simulink model "read_scaled_imu"  (R2024a)
settings: Solver=ode4  StartTime=0.0  StopTime=100  FixedStep=sampleTime  RelTol=1e-3
values from neighbouring files (symbols this model uses):
  sampleTime = 1/500    (= 0.002)    [read_imu.m]
undefined symbols (not defined in the file or in its folder): f
libraries: simulink_extras x9, uavmavlinklib x4, instrumentlib x2, aerolibanimutils x1, px4MAVLinkBridgelib x1, mspfiltlib x1, dspstat3 x1
settings Model: Creator=user  LastModifiedBy=user

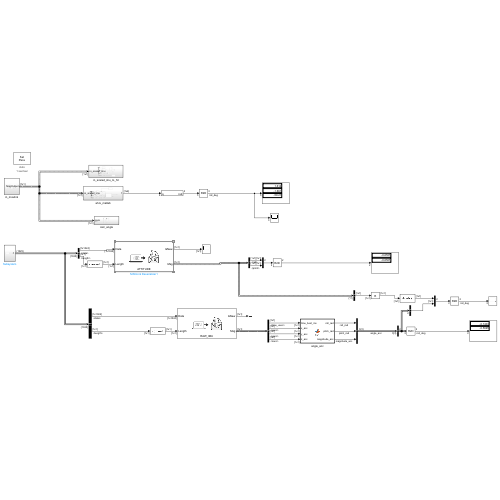
[thumbnail: Simulink's stored preview of the top-level diagram]
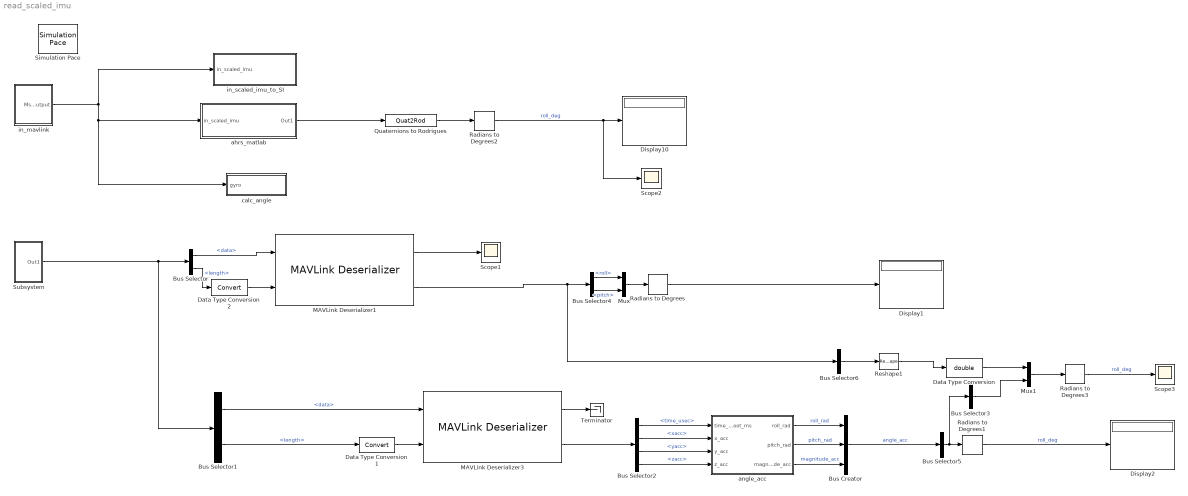
== system read_scaled_imu ==
  Bus Creator : BusCreator  Inputs=3
  Bus Selector : BusSelector  OutputSignals=data,length
  Bus Selector1 : BusSelector  OutputSignals=data,length
  Bus Selector2 : BusSelector  OutputSignals=Payload.time_usec,Payload.xacc,Payload.yacc,Payload.zacc
  Bus Selector3 : BusSelector  OutputSignals=roll_rad  OutputAsBus=on
  Bus Selector4 : BusSelector  OutputSignals=Payload.roll,Payload.pitch
  Bus Selector5 : BusSelector  OutputSignals=roll_rad,pitch_rad  OutputAsBus=on
  Bus Selector6 : BusSelector  OutputSignals=Payload.roll  OutputAsBus=on
  Data Type Conversion : DataTypeConversion  OutDataTypeStr=double  SaturateOnIntegerOverflow=off  RndMeth=Floor
  Data Type Conversion1 : DataTypeConversion  SaturateOnIntegerOverflow=off  RndMeth=Floor
  Data Type Conversion2 : DataTypeConversion  SaturateOnIntegerOverflow=off  RndMeth=Floor
  Display1 : Display
  Display10 : Display
  Display2 : Display
  MAVLink Deserializer1 : uavmavlinklib/MAVLink Deserializer  dialectSource=Select from standard MAVLink dialects  dialect=common.xml  dialectCustom=common.xml  version=2  messageType=ATTITUDE  inputDataLength=on  SystemIDFilter=off  systemID=1  ComponentIDFilter=off  componentID=1  queueMsg=off  queueMsgSize=50  dropNum=off
  MAVLink Deserializer3 : uavmavlinklib/MAVLink Deserializer  dialectSource=Select from standard MAVLink dialects  dialect=common.xml  dialectCustom=common.xml  version=2  messageType=RAW_IMU  inputDataLength=on  SystemIDFilter=off  systemID=1  ComponentIDFilter=off  componentID=1  queueMsg=off  queueMsgSize=50  dropNum=off
  Mux : Mux  Inputs=2
  Mux1 : Mux  Inputs=2
  Quaternions to Rodrigues : Quat2Rod
  Radians to Degrees{,1..3} (4 alike) : simulink_extras/Transformations/Radians to Degrees
  Reshape1 : Reshape  OutputDimensionality=Customize
  Scope1 : Scope
  Scope2 : Scope
  Scope3 : Scope
  Simulation Pace : aerolibanimutils/Simulation Pace  SimulationPace=1  SleepMode=Auto  OutputPaceError=off  SampleTime=sampleTime
  Subsystem : Subsystem
  Terminator : Terminator
  ahrs_matlab : Subsystem
  angle_acc : MATLAB Function  TreatAsAtomicUnit=on
  calc_angle : Subsystem
  in_mavlink : Subsystem
  in_scaled_imu_to_SI : Subsystem
  wires:
  Quaternions to Rodrigues/1 -> Radians to Degrees2/1
  Radians to Degrees2/1 -> Scope2/1, Display10/1  "roll_deg"
  ahrs_matlab/1(Out1) -> Quaternions to Rodrigues/1
  in_mavlink/1(MsgOutput) -> calc_angle/1(gyro), ahrs_matlab/1(in_scaled_imu), in_scaled_imu_to_SI/1(in_scaled_imu)
  Bus Selector4/1 -> Mux/1  "<roll>"
  MAVLink Deserializer1/2 -> Bus Selector6/1, Bus Selector4/1
  Data Type Conversion2/1 -> MAVLink Deserializer1/2
  MAVLink Deserializer1/1 -> Scope1/1
  Bus Selector4/2 -> Mux/2  "<pitch>"
  Mux/1 -> Radians to Degrees/1
  Radians to Degrees/1 -> Display1/1
  Bus Selector/1 -> MAVLink Deserializer1/1  "<data>"
  Bus Selector/2 -> Data Type Conversion2/1  "<length>"
  Data Type Conversion1/1 -> MAVLink Deserializer3/2
  Bus Selector1/2 -> Data Type Conversion1/1  "<length>"
  Bus Selector1/1 -> MAVLink Deserializer3/1  "<data>"
  Subsystem/1(Out1) -> Bus Selector1/1, Bus Selector/1
  angle_acc/3(magnitude_acc) -> Bus Creator/3  "magnitude_acc"
  Radians to Degrees1/1 -> Display2/1  "roll_deg"
  angle_acc/1(roll_rad) -> Bus Creator/1  "roll_rad"
  angle_acc/2(pitch_rad) -> Bus Creator/2  "pitch_rad"
  Bus Creator/1 -> Bus Selector5/1  "angle_acc"
  MAVLink Deserializer3/2 -> Bus Selector2/1
  Bus Selector2/3 -> angle_acc/3(y_acc)  "<yacc>"
  Bus Selector2/2 -> angle_acc/2(x_acc)  "<xacc>"
  Bus Selector5/1 -> Bus Selector3/1, Radians to Degrees1/1
  Bus Selector2/4 -> angle_acc/4(z_acc)  "<zacc>"
  Bus Selector2/1 -> angle_acc/1(time_boot_ms)  "<time_usec>"
  Bus Selector6/1 -> Reshape1/1
  Bus Selector3/1 -> Mux1/2
  Mux1/1 -> Radians to Degrees3/1
  Radians to Degrees3/1 -> Scope3/1  "roll_deg"
  Reshape1/1 -> Data Type Conversion/1
  Data Type Conversion/1 -> Mux1/1
  MAVLink Deserializer3/1 -> Terminator/1

== system read_scaled_imu/Subsystem ==
  Bus Creator : BusCreator  Inputs=2
  MAVLink Bridge Source : px4MAVLinkBridgelib/MAVLink Bridge Source  PixhawkSerialPorttemp=COM7  PixhawkSerialPortManually=COM4  dataLength=1024  FieldTable={ 'UDP', '127.0.0.1', '14550' }  SampleTime=1/50
  Out1 : Outport
  wires:
  MAVLink Bridge Source/2 -> Bus Creator/2  "length"
  MAVLink Bridge Source/1 -> Bus Creator/1  "data"
  Bus Creator/1 -> Out1/1

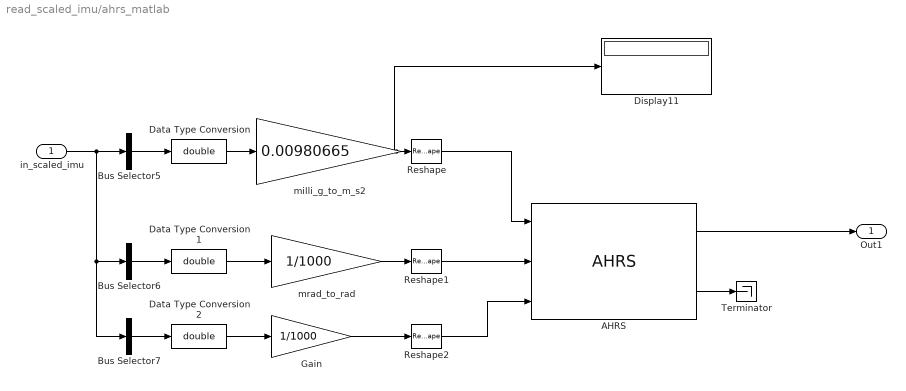
== system read_scaled_imu/ahrs_matlab ==
  in_scaled_imu : Inport
  AHRS : mspfiltlib/AHRS  DispRefFrame=ENU  DecimationFactor=1  InitialProcessNoise=ahrsfilter.defaultProcessNoise  OrientationFormat=quaternion  SimulateUsing=Code generation  AccelerometerNoise=0.0001924722*0+5.11e-6  GyroscopeNoise=9.1385e-5*0+6.86e-8  MagnetometerNoise=0.1e-5  GyroscopeDriftNoise=3.0462e-13*0+1e-8  LinearAccelerationNoise=0.0096236100000000012  MagneticDisturbanceNoise=0.5  LinearAccelerationDecayFactor=0.5*0  MagneticDisturbanceDecayFactor=0.5  ExpectedMagneticFieldStrength=50
  Bus Selector5 : BusSelector  OutputSignals=Payload.xacc,Payload.yacc,Payload.zacc  OutputAsBus=on
  Bus Selector6 : BusSelector  OutputSignals=Payload.xgyro,Payload.ygyro,Payload.zgyro  OutputAsBus=on
  Bus Selector7 : BusSelector  OutputSignals=Payload.xmag,Payload.ymag,Payload.zmag  OutputAsBus=on
  Data Type Conversion : DataTypeConversion  OutDataTypeStr=double  SaturateOnIntegerOverflow=off  RndMeth=Floor
  Data Type Conversion1 : DataTypeConversion  OutDataTypeStr=double  SaturateOnIntegerOverflow=off  RndMeth=Floor
  Data Type Conversion2 : DataTypeConversion  OutDataTypeStr=double  SaturateOnIntegerOverflow=off  RndMeth=Floor
  Display11 : Display
  Gain : Gain  Gain=1/1000
  Reshape : Reshape  OutputDimensionality=Customize  OutputDimensions=[1,3]
  Reshape1 : Reshape  OutputDimensionality=Customize  OutputDimensions=[1,3]
  Reshape2 : Reshape  OutputDimensionality=Customize  OutputDimensions=[1,3]
  Terminator : Terminator
  milli_g_to_m_s2 : Gain  Gain=0.00980665
  mrad_to_rad : Gain  Gain=1/1000
  Out1 : Outport
  wires:
  Bus Selector5/1 -> Data Type Conversion/1
  in_scaled_imu/1 -> Bus Selector6/1, Bus Selector7/1, Bus Selector5/1
  Data Type Conversion/1 -> milli_g_to_m_s2/1
  Bus Selector6/1 -> Data Type Conversion1/1
  Bus Selector7/1 -> Data Type Conversion2/1
  milli_g_to_m_s2/1 -> Display11/1, Reshape/1
  Data Type Conversion1/1 -> mrad_to_rad/1
  Reshape2/1 -> AHRS/3
  Data Type Conversion2/1 -> Gain/1
  mrad_to_rad/1 -> Reshape1/1
  Reshape1/1 -> AHRS/2
  Gain/1 -> Reshape2/1
  Reshape/1 -> AHRS/1
  AHRS/1 -> Out1/1
  AHRS/2 -> Terminator/1

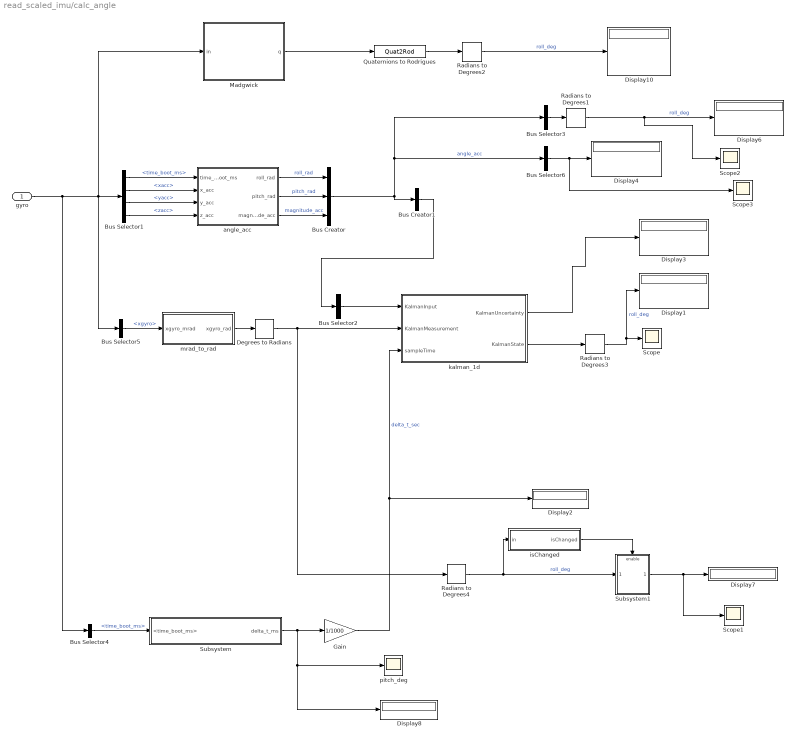
== system read_scaled_imu/calc_angle ==
  gyro : Inport
  Bus Creator : BusCreator  Inputs=3
  Bus Creator1 : BusCreator  Inputs=1
  Bus Selector1 : BusSelector  OutputSignals=Payload.time_boot_ms,Payload.xacc,Payload.yacc,Payload.zacc
  Bus Selector2 : BusSelector  OutputSignals=angle_acc.roll_rad  OutputAsBus=on
  Bus Selector3 : BusSelector  OutputSignals=roll_rad,pitch_rad  OutputAsBus=on
  Bus Selector4 : BusSelector  OutputSignals=Payload.time_boot_ms
  Bus Selector5 : BusSelector  OutputSignals=Payload.xgyro
  Bus Selector6 : BusSelector  OutputSignals=magnitude_acc  OutputAsBus=on
  Degrees to Radians : simulink_extras/Transformations/Degrees to Radians
  Display{1..4,6..8,10} (8 alike) : Display
  Gain : Gain  Gain=1/1000
  Madgwick : Subsystem
  Quaternions to Rodrigues : Quat2Rod
  Radians to Degrees{1..4} (4 alike) : simulink_extras/Transformations/Radians to Degrees
  Scope{,1..3} (4 alike) : Scope
  Subsystem : Subsystem
  Subsystem1 : Subsystem
  angle_acc : MATLAB Function  TreatAsAtomicUnit=on
  isChanged : Subsystem
  kalman_1d : Subsystem
  mrad_to_rad : Subsystem
  pitch_deg : Scope
  wires:
  Subsystem/1(delta_t_ms) -> Gain/1, Display8/1, pitch_deg/1
  Radians to Degrees3/1 -> Display1/1, Scope/1  "roll_deg"
  Bus Selector1/3 -> angle_acc/3(y_acc)  "<yacc>"
  Bus Selector1/2 -> angle_acc/2(x_acc)  "<xacc>"
  gyro/1 -> Bus Selector5/1, Madgwick/1(in), Bus Selector1/1, Bus Selector4/1
  Radians to Degrees4/1 -> Subsystem1/1(roll_deg), isChanged/1(in)  "roll_deg"
  Bus Selector3/1 -> Radians to Degrees1/1
  Gain/1 -> Display2/1, kalman_1d/3(sampleTime)  "delta_t_sec"
  Bus Creator/1 -> Bus Creator1/1, Bus Selector6/1, Bus Selector3/1  "angle_acc"
  Bus Selector1/1 -> angle_acc/1(time_boot_ms)  "<time_boot_ms>"
  Bus Selector1/4 -> angle_acc/4(z_acc)  "<zacc>"
  angle_acc/2(pitch_rad) -> Bus Creator/2  "pitch_rad"
  Bus Selector4/1 -> Subsystem/1(<time_boot_ms>)  "<time_boot_ms>"
  angle_acc/1(roll_rad) -> Bus Creator/1  "roll_rad"
  Bus Creator1/1 -> Bus Selector2/1
  Bus Selector5/1 -> mrad_to_rad/1(xgyro_mrad)  "<xgyro>"
  mrad_to_rad/1(xgyro_rad) -> Degrees to Radians/1
  Subsystem1/1(Out1) -> Scope1/1, Display7/1
  isChanged/1(isChanged) -> Subsystem1/Enable
  Bus Selector2/1 -> kalman_1d/1(KalmanInput)
  kalman_1d/1(KalmanUncertainty) -> Display3/1
  kalman_1d/2(KalmanState) -> Radians to Degrees3/1
  Degrees to Radians/1 -> Radians to Degrees4/1, kalman_1d/2(KalmanMeasurement)
  Radians to Degrees2/1 -> Display10/1  "roll_deg"
  Madgwick/1(q) -> Quaternions to Rodrigues/1
  Quaternions to Rodrigues/1 -> Radians to Degrees2/1
  Radians to Degrees1/1 -> Scope2/1, Display6/1  "roll_deg"
  angle_acc/3(magnitude_acc) -> Bus Creator/3  "magnitude_acc"
  Bus Selector6/1 -> Scope3/1, Display4/1

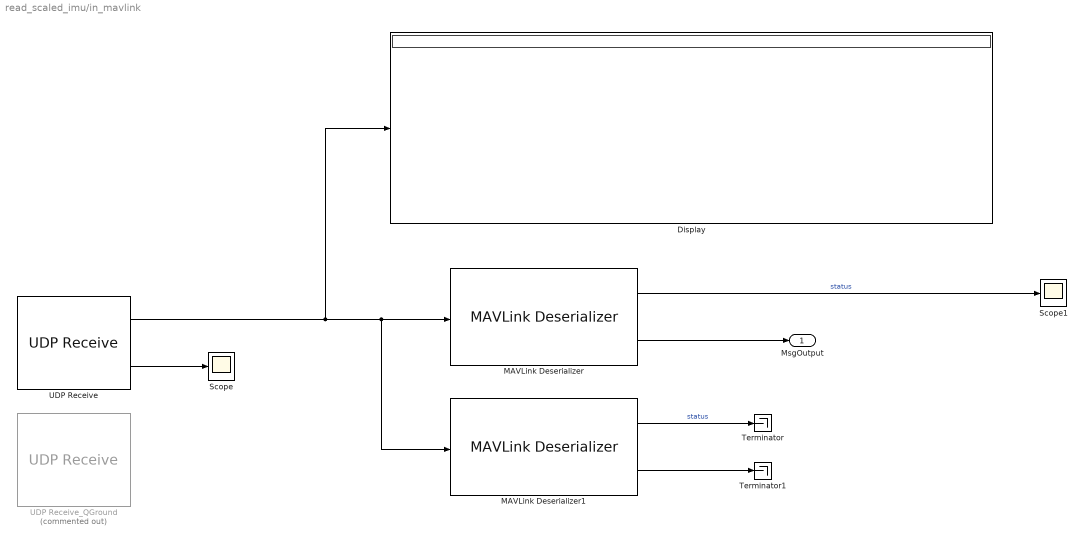
== system read_scaled_imu/in_mavlink ==
  Display : Display
  MAVLink Deserializer : uavmavlinklib/MAVLink Deserializer  dialectSource=Select from standard MAVLink dialects  dialect=common.xml  dialectCustom=common.xml  version=2  messageType=SCALED_IMU  inputDataLength=off  SystemIDFilter=off  systemID=1  ComponentIDFilter=off  componentID=1  queueMsg=off  queueMsgSize=50  dropNum=off
  MAVLink Deserializer1 : uavmavlinklib/MAVLink Deserializer  dialectSource=Select from standard MAVLink dialects  dialect=common.xml  dialectCustom=common.xml  version=2  messageType=HEARTBEAT  inputDataLength=off  SystemIDFilter=off  systemID=1  ComponentIDFilter=off  componentID=1  queueMsg=off  queueMsgSize=50  dropNum=off
  Scope : Scope
  Scope1 : Scope
  Terminator : Terminator
  Terminator1 : Terminator
  UDP Receive : instrumentlib/UDP Receive  LocalAddress=192.168.137.1  LocalPort=14550  EnablePortSharing=on  Host=127.0.0.1  Port=14550  GetLatestData=off  DataSize=100  DataType=uint8  ASCIIFormatting=%f,  Terminator=LF  CustomTerminator=10  ByteOrder=big-endian  EnableBlockingMode=off  Timeout=10  SampleTime=-1  SimulateUsing=Interpreted execution
  UDP Receive_QGround : instrumentlib/UDP Receive  Commented=on  LocalAddress=localhost  LocalPort=14445  EnablePortSharing=on  Host=127.0.0.1  Port=14550  GetLatestData=off  DataSize=256  DataType=uint8  ASCIIFormatting=%f,  Terminator=LF  CustomTerminator=10  ByteOrder=big-endian  EnableBlockingMode=off  Timeout=10  SampleTime=-1  SimulateUsing=Interpreted execution
  MsgOutput : Outport
  wires:
  MAVLink Deserializer/1 -> Scope1/1  "status"
  UDP Receive/1 -> Display/1, MAVLink Deserializer1/1, MAVLink Deserializer/1
  UDP Receive/2 -> Scope/1
  MAVLink Deserializer/2 -> MsgOutput/1
  MAVLink Deserializer1/1 -> Terminator/1  "status"
  MAVLink Deserializer1/2 -> Terminator1/1

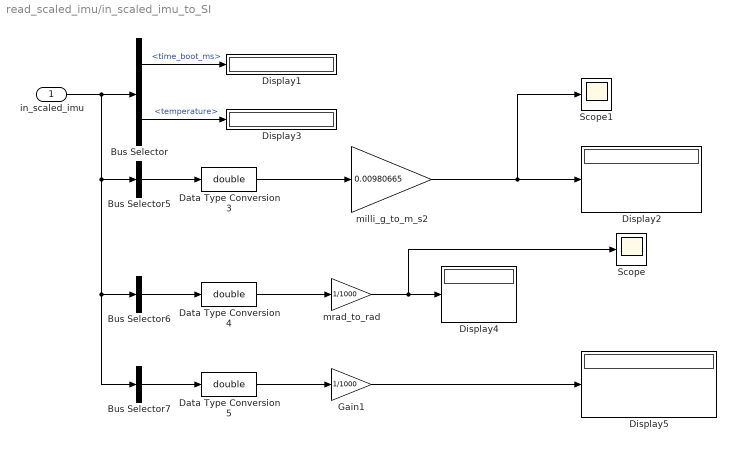
== system read_scaled_imu/in_scaled_imu_to_SI ==
  in_scaled_imu : Inport
  Bus Selector : BusSelector  OutputSignals=Payload.time_boot_ms,Payload.temperature
  Bus Selector5 : BusSelector  OutputSignals=Payload.xacc,Payload.yacc,Payload.zacc  OutputAsBus=on
  Bus Selector6 : BusSelector  OutputSignals=Payload.xgyro,Payload.ygyro,Payload.zgyro  OutputAsBus=on
  Bus Selector7 : BusSelector  OutputSignals=Payload.xmag,Payload.ymag,Payload.zmag  OutputAsBus=on
  Data Type Conversion3 : DataTypeConversion  OutDataTypeStr=double  SaturateOnIntegerOverflow=off  RndMeth=Floor
  Data Type Conversion4 : DataTypeConversion  OutDataTypeStr=double  SaturateOnIntegerOverflow=off  RndMeth=Floor
  Data Type Conversion5 : DataTypeConversion  OutDataTypeStr=double  SaturateOnIntegerOverflow=off  RndMeth=Floor
  Display{1..5} (5 alike) : Display
  Gain1 : Gain  Gain=1/1000
  Scope : Scope
  Scope1 : Scope
  milli_g_to_m_s2 : Gain  Gain=0.00980665
  mrad_to_rad : Gain  Gain=1/1000
  wires:
  Bus Selector/1 -> Display1/1  "<time_boot_ms>"
  in_scaled_imu/1 -> Bus Selector7/1, Bus Selector6/1, Bus Selector5/1, Bus Selector/1
  Bus Selector/2 -> Display3/1  "<temperature>"
  Bus Selector7/1 -> Data Type Conversion5/1
  Data Type Conversion5/1 -> Gain1/1
  Bus Selector6/1 -> Data Type Conversion4/1
  Data Type Conversion4/1 -> mrad_to_rad/1
  Bus Selector5/1 -> Data Type Conversion3/1
  Data Type Conversion3/1 -> milli_g_to_m_s2/1
  Gain1/1 -> Display5/1
  mrad_to_rad/1 -> Scope/1, Display4/1
  milli_g_to_m_s2/1 -> Scope1/1, Display2/1

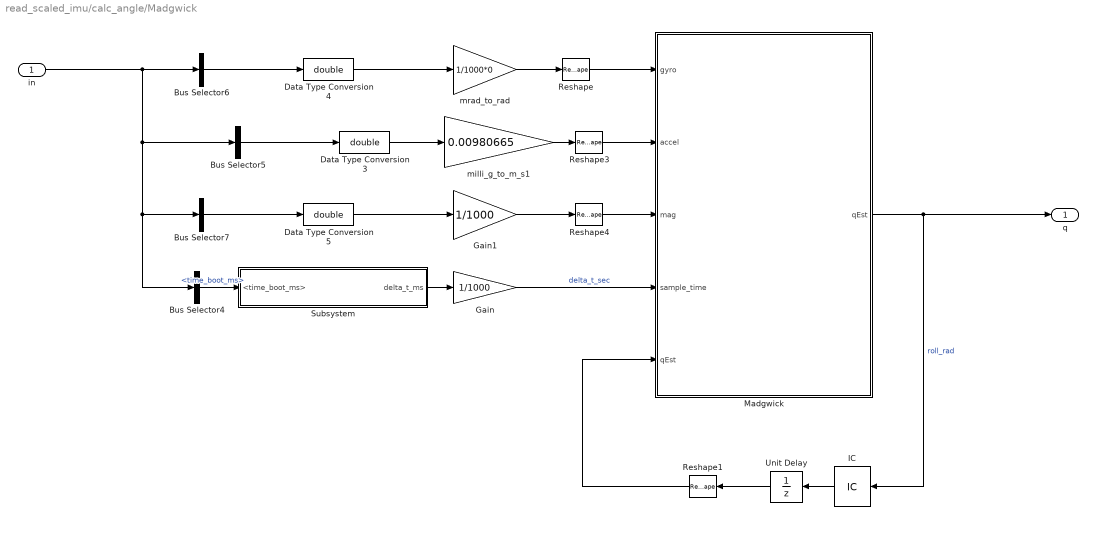
== system read_scaled_imu/calc_angle/Madgwick ==
  in : Inport
  Bus Selector4 : BusSelector  OutputSignals=Payload.time_boot_ms
  Bus Selector5 : BusSelector  OutputSignals=Payload.xacc,Payload.yacc,Payload.zacc  OutputAsBus=on
  Bus Selector6 : BusSelector  OutputSignals=Payload.xgyro,Payload.ygyro,Payload.zgyro  OutputAsBus=on
  Bus Selector7 : BusSelector  OutputSignals=Payload.xmag,Payload.ymag,Payload.zmag  OutputAsBus=on
  Data Type Conversion3 : DataTypeConversion  OutDataTypeStr=double  SaturateOnIntegerOverflow=off  RndMeth=Floor
  Data Type Conversion4 : DataTypeConversion  OutDataTypeStr=double  SaturateOnIntegerOverflow=off  RndMeth=Floor
  Data Type Conversion5 : DataTypeConversion  OutDataTypeStr=double  SaturateOnIntegerOverflow=off  RndMeth=Floor
  Gain : Gain  Gain=1/1000
  Gain1 : Gain  Gain=1/1000
  IC : InitialCondition  Value=[1 0 0 0]
  Madgwick : MATLAB Function  TreatAsAtomicUnit=on
  Reshape : Reshape  OutputDimensionality=Customize  OutputDimensions=[1,3]
  Reshape1 : Reshape  OutputDimensionality=Customize  OutputDimensions=[1,4]
  Reshape3 : Reshape  OutputDimensionality=Customize  OutputDimensions=[1,3]
  Reshape4 : Reshape  OutputDimensionality=Customize  OutputDimensions=[1,3]
  Subsystem : Subsystem
  Unit Delay : UnitDelay  SampleTime=-1  HasFrameUpgradeWarning=on
  milli_g_to_m_s1 : Gain  Gain=0.00980665
  mrad_to_rad : Gain  Gain=1/1000*0
  q : Outport
  wires:
  in/1 -> Bus Selector4/1, Bus Selector7/1, Bus Selector5/1, Bus Selector6/1
  Bus Selector6/1 -> Data Type Conversion4/1
  Bus Selector7/1 -> Data Type Conversion5/1
  Bus Selector5/1 -> Data Type Conversion3/1
  Gain1/1 -> Reshape4/1
  Bus Selector4/1 -> Subsystem/1(<time_boot_ms>)  "<time_boot_ms>"
  Data Type Conversion5/1 -> Gain1/1
  Data Type Conversion4/1 -> mrad_to_rad/1
  Data Type Conversion3/1 -> milli_g_to_m_s1/1
  Subsystem/1(delta_t_ms) -> Gain/1
  mrad_to_rad/1 -> Reshape/1
  milli_g_to_m_s1/1 -> Reshape3/1
  Gain/1 -> Madgwick/4(sample_time)  "delta_t_sec"
  Madgwick/1(qEst) -> IC/1, q/1  "roll_rad"
  Reshape/1 -> Madgwick/1(gyro)
  Reshape3/1 -> Madgwick/2(accel)
  Reshape4/1 -> Madgwick/3(mag)
  Reshape1/1 -> Madgwick/5("qEst ")
  Unit Delay/1 -> Reshape1/1
  IC/1 -> Unit Delay/1

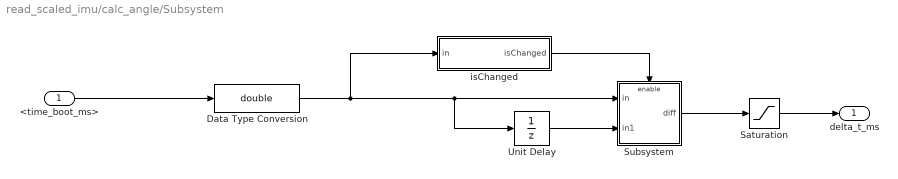
== system read_scaled_imu/calc_angle/Subsystem ==
  <time_boot_ms> : Inport
  Data Type Conversion : DataTypeConversion  OutDataTypeStr=double  SaturateOnIntegerOverflow=off  RndMeth=Floor
  Saturation : Saturate  UpperLimit=1000  LowerLimit=0
  Subsystem : Subsystem
  Unit Delay : UnitDelay  SampleTime=-1  HasFrameUpgradeWarning=on
  isChanged : Subsystem
  delta_t_ms : Outport
  wires:
  <time_boot_ms>/1 -> Data Type Conversion/1
  isChanged/1(isChanged) -> Subsystem/Enable
  Unit Delay/1 -> Subsystem/2(in1)
  Subsystem/1(diff) -> Saturation/1
  Data Type Conversion/1 -> isChanged/1(in), Unit Delay/1, Subsystem/1(in)
  Saturation/1 -> delta_t_ms/1

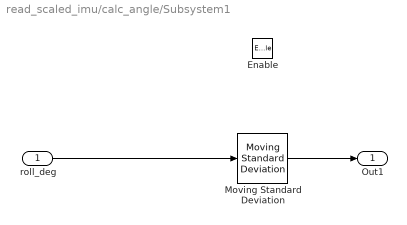
== system read_scaled_imu/calc_angle/Subsystem1 ==
  roll_deg : Inport
  Enable : EnablePort
  Moving Standard Deviation : dspstat3/Moving Standard Deviation  Method=Sliding window  ForgettingFactorPort=off  SpecifyWindowLength=on  WindowLength=10  OverlapLength=9  AllowArbitraryInputLength=off  ForgettingFactor=0.9  SimulateUsing=Interpreted execution
  Out1 : Outport
  wires:
  Moving Standard Deviation/1 -> Out1/1
  roll_deg/1 -> Moving Standard Deviation/1

== system read_scaled_imu/calc_angle/isChanged ==
  in : Inport
  Equal : RelationalOperator  Operator=~=  OutDataTypeStr=boolean  RndMeth=Simplest  InputSameDT=off
  Unit Delay : UnitDelay  SampleTime=-1  HasFrameUpgradeWarning=on
  isChanged : Outport
  wires:
  in/1 -> Equal/2, Unit Delay/1
  Unit Delay/1 -> Equal/1
  Equal/1 -> isChanged/1

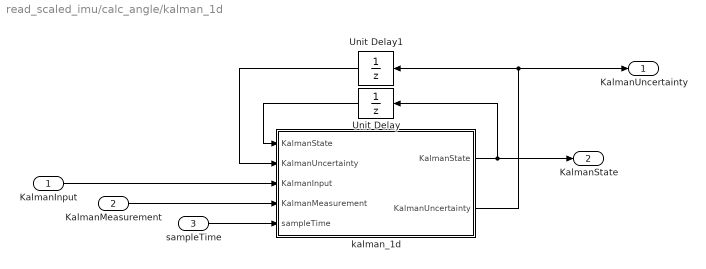
== system read_scaled_imu/calc_angle/kalman_1d ==
  KalmanInput : Inport
  KalmanMeasurement : Inport  Port=2
  sampleTime : Inport  Port=3
  Unit Delay : UnitDelay  SampleTime=-1  HasFrameUpgradeWarning=on
  Unit Delay1 : UnitDelay  SampleTime=-1  HasFrameUpgradeWarning=on
  kalman_1d : MATLAB Function  TreatAsAtomicUnit=on
  KalmanUncertainty : Outport
  KalmanState : Outport  Port=2
  wires:
  KalmanMeasurement/1 -> kalman_1d/4(KalmanMeasurement)
  kalman_1d/2(KalmanUncertainty) -> KalmanUncertainty/1, Unit Delay1/1
  sampleTime/1 -> kalman_1d/5(sampleTime)
  kalman_1d/1(KalmanState) -> KalmanState/1, Unit Delay/1
  Unit Delay1/1 -> kalman_1d/2("KalmanUncertainty ")
  KalmanInput/1 -> kalman_1d/3(KalmanInput)
  Unit Delay/1 -> kalman_1d/1("KalmanState ")

== system read_scaled_imu/calc_angle/mrad_to_rad ==
  xgyro_mrad : Inport
  Data Type Conversion4 : DataTypeConversion  OutDataTypeStr=double  SaturateOnIntegerOverflow=off  RndMeth=Floor
  mrad_to_rad : Gain  Gain=1/1000
  xgyro_rad : Outport
  wires:
  Data Type Conversion4/1 -> mrad_to_rad/1
  xgyro_mrad/1 -> Data Type Conversion4/1
  mrad_to_rad/1 -> xgyro_rad/1

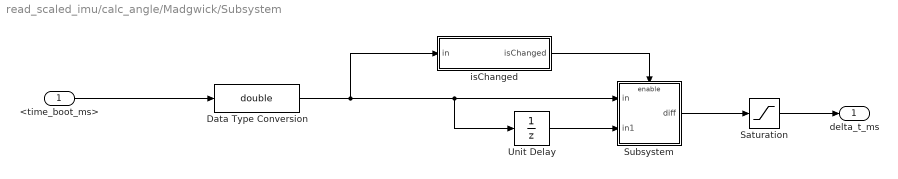
== system read_scaled_imu/calc_angle/Madgwick/Subsystem ==
  <time_boot_ms> : Inport
  Data Type Conversion : DataTypeConversion  OutDataTypeStr=double  SaturateOnIntegerOverflow=off  RndMeth=Floor
  Saturation : Saturate  UpperLimit=1000  LowerLimit=0
  Subsystem : Subsystem
  Unit Delay : UnitDelay  SampleTime=-1  HasFrameUpgradeWarning=on
  isChanged : Subsystem
  delta_t_ms : Outport
  wires:
  <time_boot_ms>/1 -> Data Type Conversion/1
  isChanged/1(isChanged) -> Subsystem/Enable
  Unit Delay/1 -> Subsystem/2(in1)
  Subsystem/1(diff) -> Saturation/1
  Data Type Conversion/1 -> isChanged/1(in), Unit Delay/1, Subsystem/1(in)
  Saturation/1 -> delta_t_ms/1

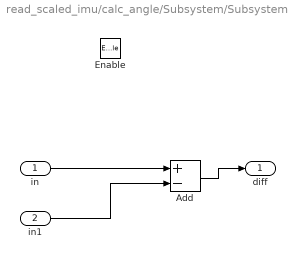
== system read_scaled_imu/calc_angle/Subsystem/Subsystem ==
  in : Inport
  in1 : Inport  Port=2
  Enable : EnablePort
  Add : Sum  Inputs=+-
  diff : Outport
  wires:
  Add/1 -> diff/1
  in/1 -> Add/1
  in1/1 -> Add/2

== system read_scaled_imu/calc_angle/Subsystem/isChanged ==
  in : Inport
  Equal : RelationalOperator  Operator=~=  OutDataTypeStr=boolean  RndMeth=Simplest  InputSameDT=off
  Unit Delay : UnitDelay  SampleTime=-1  HasFrameUpgradeWarning=on
  isChanged : Outport
  wires:
  in/1 -> Equal/2, Unit Delay/1
  Unit Delay/1 -> Equal/1
  Equal/1 -> isChanged/1

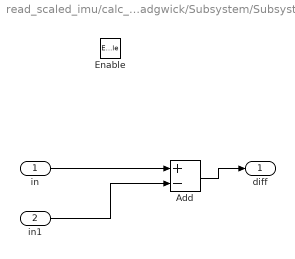
== system read_scaled_imu/calc_angle/Madgwick/Subsystem/Subsystem ==
  in : Inport
  in1 : Inport  Port=2
  Enable : EnablePort
  Add : Sum  Inputs=+-
  diff : Outport
  wires:
  Add/1 -> diff/1
  in/1 -> Add/1
  in1/1 -> Add/2

== system read_scaled_imu/calc_angle/Madgwick/Subsystem/isChanged ==
  in : Inport
  Equal : RelationalOperator  Operator=~=  OutDataTypeStr=boolean  RndMeth=Simplest  InputSameDT=off
  Unit Delay : UnitDelay  SampleTime=-1  HasFrameUpgradeWarning=on
  isChanged : Outport
  wires:
  in/1 -> Equal/2, Unit Delay/1
  Unit Delay/1 -> Equal/1
  Equal/1 -> isChanged/1

== matlab function read_scaled_imu/calc_angle/kalman_1d/kalman_1d ==
  data: KalmanState input; KalmanState output; KalmanUncertainty input; KalmanInput input; KalmanMeasurement input; KalmanUncertainty output; sampleTime input
% https://www.youtube.com/watch?v=5HuN9iL-zxU&list=PLeuMA6tJBPKsAfRfFuGrEljpBow5hPVD4&index=18&ab_channel=CarbonAeronautics

function [KalmanState,KalmanUncertainty]  = fcn(KalmanState, KalmanUncertainty, KalmanInput, KalmanMeasurement,sampleTime)
% float KalmanAngleRoll=0, KalmanUncertaintyAngleRoll=2*2;
% float KalmanAnglePitch=0, KalmanUncertaintyAnglePitch=2*2;
% float Kalman1DOutput[]={0,0};

% KalmanState : angle calculated with Kalman Filter
% KalmanInput : rotation  rate (rad/sec)
% Kalman  Measurement : Acceleroemeter angle

std_deviation_rate = deg2rad(1.5);
std_deviation_KalmanUncertainty =  deg2rad(1);

% Predict the  current state of the system
KalmanState=KalmanState+sampleTime*KalmanInput;
% Calculate  the uncertainty  of the prediction
KalmanUncertainty=KalmanUncertainty + sampleTime * sampleTime * std_deviation_rate * std_deviation_rate;
% Calculate KalmanGainfrom  uncreatrinities on predictions and measurements
KalmanGain=KalmanUncertainty * 1/(1*KalmanUncertainty + std_deviation_KalmanUncertainty * std_deviation_KalmanUncertainty);
% Update the predicrted stat oftje system with the measurement of the state
KalmanState=KalmanState+KalmanGain * (KalmanMeasurement-KalmanState);
KalmanUncertainty=(1-KalmanGain) * KalmanUncertainty;

== matlab function read_scaled_imu/calc_angle/angle_acc ==
  data: time_boot_ms input; roll_rad output; x_acc input; y_acc input; z_acc input; pitch_rad output; magnitude_acc output
%% References : https://www.youtube.com/watch?v=7VW_XVbtu9k&list=PLeuMA6tJBPKsAfRfFuGrEljpBow5hPVD4&index=17&ab_channel=CarbonAeronautics

function [roll_rad,pitch_rad,magnitude_acc] = fcn(time_boot_ms,x_acc,y_acc,z_acc)

persistent roll_rad_pre pitch_rad_pre
if(isempty(roll_rad_pre))
roll_rad_pre = 0;
pitch_rad_pre = 0;
end

x_acc = double(x_acc);
y_acc = double(y_acc);
z_acc = double(z_acc);

%% acc update only if acc in range 0.9g - 1.1g
magnitude_acc = sqrt(x_acc*x_acc + y_acc*y_acc + z_acc*z_acc)/1000;
percent = 7.5/100;
if(magnitude_acc < (1+percent) && magnitude_acc > (1-percent))

roll_rad_calculated = atan(-y_acc/sqrt((x_acc*x_acc)+(z_acc*z_acc)));
pitch_rad_calculated = atan(x_acc/sqrt((y_acc*y_acc)+(z_acc*z_acc)));

roll_rad_pre = roll_rad_calculated;
pitch_rad_pre = pitch_rad_calculated;

else

end

roll_rad = roll_rad_pre;
pitch_rad = pitch_rad_pre;

end

== matlab function read_scaled_imu/calc_angle/Madgwick/Madgwick ==
  data: gyro input; qEst output; accel input; mag input; sample_time input; qEst input


%  Refeences : https://www.olliw.eu/2013/imu-data-fusing/
% https://github.com/memsindustrygroup/Open-Source-Sensor-Fusion/tree/master/docs

function qEst  = fcn(gyro, accel, mag, sample_time,qEst)
%% Madgwick Filter Implementation
%  Source: https://x-io.co.uk/open-source-imu-and-ahrs-algorithms/

% persistent qEst
% if isempty(qEst)
%     qEst = [1; 0; 0; 0]; % Initial orientation quaternion
% end

updateFreq = 1/sample_time;          % frequency at which filter is updated
beta = 0.1;                % represents mean zero gyro measurement error
zeta = 0;                  % gain used for gyro bias drift compensation


% update() should be called at the filter's update frequency
% gyro = [gx gy gz]
% accel = [ax ay az]
% mag = [mx my mz]

% put IMU measurements in 4D arrays
gyro = [0 gyro];
accel = [0 accel];
mag = [0 mag];

% for convenience
q = qEst;

% angular rate quaternion
qDot = 0.5 * [q(1)*gyro(1) - q(2)*gyro(2) - q(3)*gyro(3) - q(4)*gyro(4);
    q(1)*gyro(2) + q(2)*gyro(1) + q(3)*gyro(4) - q(4)*gyro(3);
    q(1)*gyro(3) - q(2)*gyro(4) + q(3)*gyro(1) + q(4)*gyro(2);
    q(1)*gyro(4) + q(2)*gyro(3) - q(3)*gyro(2) + q(4)*gyro(1)]';

% only compute feedback if accelerometer values are valid, (avoid Nan)
if any(accel)
    % normalize accel measurement
    accel = accel / norm(accel);

    % objective function: fg(q, a) = q*g*q' - a (where g = [0 0 0 1])
    fg = 2 * [q(2)*q(4) - q(1)*q(3) - accel(2);
        q(1)*q(2) + q(3)*q(4) - accel(3);
        0.5 - q(2)^2 - q(3)^2 - accel(4)];

    % jacobian: Jg(q)
    jg = 2 * [-q(3),  q(2),   0;
        q(4),  q(1),  -2*q(2);
        -q(1),  q(4),  -2*q(3);
        q(2),  q(3),   0];

    % function gradient = Jg(q)fg(q, a)
    gradient = (jg * fg)';

    % only use magnetometer measurement if it is valid (avoid NaN)
    if any(mag)
        % normalize mag measurement
        mag = mag / norm(mag);

        % measured direction of Earth's magnetic field in earth frame
        % h = q*mag*q' (quaternion rotation)
        h = [0;
            2*q(1)*(q(2)*mag(1) + q(3)*mag(4) - q(4)*mag(3)) + mag(2)*(q(1)^2 - q(2)^2 - q(3)^2 - q(4)^2);
            2*(mag(2)*(q(1)*q(4) + q(2)*q(3)) + mag(4)*(q(3)*q(4) - q(1)*q(2))) + mag(3)*(q(1)^2 - q(2)^2 + q(3)^2 - q(4)^2);
            2*(mag(2)*(q(2)*q(4) - q(1)*q(3)) + mag(3)*(q(1)*q(2) + q(3)*q(4))) + mag(4)*(q(1)^2 - q(2)^2 - q(3)^2 + q(4)^2)]';

        % compensate for magnetic distortions
        b = [0, sqrt(h(2)^2 + h(3)^2), 0, h(4)];

        % objective function: fb(q, b, m) = q*b*q' - m
        fb = [2*b(2)*(0.5 - q(3)^2 - q(4)^2) + 2*b(4)*(q(2)*q(4) - q(1)*q(3)) - mag(2);
            2*b(2)*(q(2)*q(3) - q(1)*q(4)) + 2*b(4)*(q(1)*q(2) + q(3)*q(4)) - mag(3);
            2*b(2)*(q(1)*q(3) + q(2)*q(4)) + 2*b(4)*(0.5 - q(2)^2 - q(3)^2) - mag(4)];

        % jacobian: J(q, b)
        jb = 2 * [-b(4)*q(3),                -b(2)*q(4) + b(4)*q(2),  b(2)*q(3);
            b(4)*q(4),                 b(2)*q(3) + b(4)*q(1),  b(2)*q(4) - 2*b(4)*q(2);
            -2*b(2)*q(3) - b(4)*q(1),   b(2)*q(2) + b(4)*q(4),  b(2)*q(1) - 2*b(4)*q(3);
            -2*b(2)*q(4) + b(4)*q(2),  -b(2)*q(1) + b(4)*q(4),  b(2)*q(2)];

        % function gradient = Jgb(q)fgb(q, a, b, m)
        gradient = gradient + (jb * fb)';
    end

    % normalize gradient
    if any(gradient)
        gradient = gradient / norm(gradient);
    end

    % compensate for gyro bias drift
    gyroErr = 2 * [q(1)*gradient(1) + q(2)*gradient(2) + q(3)*gradient(3) + q(4)*gradient(4);
        q(1)*gradient(2) - q(2)*gradient(1) - q(3)*gradient(4) + q(4)*gradient(3);
        q(1)*gradient(3) + q(2)*gradient(4) - q(3)*gradient(1) - q(4)*gradient(2);
        q(1)*gradient(4) - q(2)*gradient(3) + q(3)*gradient(2) - q(4)*gradient(1)]';

    % integrate
    gyroBias = gyroErr / updateFreq * zeta;

    % compute compesnated gyro measurement
    gyro = gyro - gyroBias;

    % recompute angular rate quaternion
    qDot = 0.5 * [q(1)*gyro(1) - q(2)*gyro(2) - q(3)*gyro(3) - q(4)*gyro(4);
        q(1)*gyro(2) + q(2)*gyro(1) + q(3)*gyro(4) - q(4)*gyro(3);
        q(1)*gyro(3) - q(2)*gyro(4) + q(3)*gyro(1) + q(4)*gyro(2);
        q(1)*gyro(4) + q(2)*gyro(3) - q(3)*gyro(2) + q(4)*gyro(1)]';

    % apply feedback
    qDot = qDot - beta * gradient;
end

% integrate rate of change and add to current quaternion
qEst = qEst + qDot / updateFreq;
if any(qEst)
    qEst = qEst / norm(qEst);
end
end

== matlab function read_scaled_imu/angle_acc ==
  data: time_boot_ms input; roll_rad output; x_acc input; y_acc input; z_acc input; pitch_rad output; magnitude_acc output
%% References : https://www.youtube.com/watch?v=7VW_XVbtu9k&list=PLeuMA6tJBPKsAfRfFuGrEljpBow5hPVD4&index=17&ab_channel=CarbonAeronautics

function [roll_rad,pitch_rad,magnitude_acc] = fcn(time_boot_ms,x_acc,y_acc,z_acc)

persistent roll_rad_pre pitch_rad_pre
if(isempty(roll_rad_pre))
roll_rad_pre = 0;
pitch_rad_pre = 0;
end

x_acc = double(x_acc);
y_acc = double(y_acc);
z_acc = double(z_acc);

%% acc update only if acc in range 0.9g - 1.1g
magnitude_acc = sqrt(x_acc*x_acc + y_acc*y_acc + z_acc*z_acc)/1000;
percent = 7.5/100;
if(magnitude_acc < (1+percent) && magnitude_acc > (1-percent))

roll_rad_calculated = atan(-y_acc/sqrt((x_acc*x_acc)+(z_acc*z_acc)));
pitch_rad_calculated = atan(x_acc/sqrt((y_acc*y_acc)+(z_acc*z_acc)));

roll_rad_pre = roll_rad_calculated;
pitch_rad_pre = pitch_rad_calculated;

else

end

roll_rad = roll_rad_pre;
pitch_rad = pitch_rad_pre;

end
